simulink model "I_PD_real_ideal"  (R2018a)
settings: Solver=FixedStepAuto  StartTime=0.0  StopTime=80  RelTol=1e-3
PreLoadFcn:
  | % Parámetros de la planta
  | K0=0.82/0.017;
  | tau0=0.26;
  | N=9;
  | Kpot=1.62;
  | % Periodo de muestreo
  | Ts=0.01;
  | % Especificaciones de control deseadas
  | Sp=80; % sobreimpulso
  | Fd=0.5; % frecuencia
  | % Polos de segundo orden continuo que cumplirán las especificaciones
  | wd=2*pi*Fd ;
  | xi=sqrt((log(Sp/100))^2/(pi^2+log(Sp/100)^2))
  | wn=wd/ sqrt(1-xi^2)
  | s1=-xi*wn+j*wd
  | s2=-xi*wn-j*wd
  | % Polos de segundo orden discreto que cumpliran las especificaciones
  | p1=exp(Ts* s1 )
  | p2=exp(Ts* s2 )
  | % Insertar el tercer y cuarto polo (no dominantes)
  | p3=0.8
  | p4=0.8
  | % Función de transferencia discreta de la planta
  | Ptas=tf([K0*(1/N)*Kpot],[tau0,1,0]);
  | Ptaz=c2d(Ptas,Ts,'zoh');
  | % Coeficientes del denominador y enumerador
  | [Nz ,Dz]= tfdata(Ptaz,'v')
  | a1=Nz(2);
  | a0=Nz(3);
  | b1=Dz(2);
  | b0=Dz(3);
  | % Definiciones de las matrices A y B
  | A=[1 a1 0 0; ...
  |    b1-1 a0 a1 0;
  |    b0-b1 0 a0 a1;
  |   -b0 0 0 a0] ;
  | b=[-b1+1-p1-p2-p3-p4;
  |    -b0+b1+p1*p2-(-p1-p2)*p3-(-p1-p2-p3)*p4;
  |    b0-p1*p2*p3-(p1*p2-(-p1-p2)*p3)*p4;
  |    p1*p2*p3*p4] ;
  | % Controlador
  | x=inv(A)*b ;
  | alpha=x(1)
  | c2=x(2)
  | c1=x(3)
  | c0=x(4)
  | A2=[1 1 1; alpha-1 alpha+1 -2; -alpha alpha 1];
  | B2=[c2;c1;c0];
  | x2=inv(A2)*B2;
  | kp = x2(1)
  | ki = (2/Ts)*x2(2)
  | kd = Ts*x2(3)
undefined symbols (not defined in the file or in its folder): DiscIntNeverNeededParam
libraries: arduinolib x4, simulink x1
settings Model: SimulationMode=external  ExtModeTrigDuration=2  Creator=Eneko Lerma  LastModifiedBy=Eneko Lerma
settings SolverCC: AutoInsertRateTranBlk=on
settings OptimizationCC: EnhancedBackFolding=on  PassReuseOutputArgsAs=Individual arguments  MaxStackSize=64  OptimizeBlockOrder=speed  DifferentSizesBufferReuse=on  OptimizationCustomize=off
settings DebuggingCC: ParameterTunabilityLossMsg=error
settings HardwareCC: ProdBitPerPointer=32  ProdBitPerSizeT=32  ProdBitPerPtrDiffT=32  ProdLargestAtomicInteger=Long  ProdLargestAtomicFloat=Double  ProdWordSize=32  ProdHWDeviceType=ARM Compatible->ARM Cortex
settings SFSimCC: MATLABDynamicMemAlloc=off
settings RTWCC: SystemTargetFile=ert.tlc  HardwareBoard=Arduino Due  TLCOptions=-aInlineSetEventsForThisBaseRateFcn=TLC_FALSE -aSuppressMultiTaskScheduler=TLC_FALSE -aRateBasedStepFcn=1  TemplateMakefile=ert_default_tmf  GenerateReport=on  Toolchain=Arduino ARM  BuildConfiguration=Faster Runs  IncludeHyperlinkInReport=on  LaunchReport=on  GenerateTraceInfo=on  GenerateTraceReport=on  GenerateTraceReportSl=on  GenerateTraceReportSf=on  GenerateTraceReportEml=on
settings RTWCC: CustomTerminator=|
  | writeDigitalPin((uint8_T)3, 0);
  | writeDigitalPin((uint8_T)5, 0);
settings CodeAppCC: ForceParamTrailComments=on  IgnoreCustomStorageClasses=off  OperatorAnnotations=on  SimulinkDataObjDesc=on  SFDataObjDesc=on  InsertBlockDesc=on
settings ERTTargetCC: SupportContinuousTime=on  SupportVariableSizeSignals=on

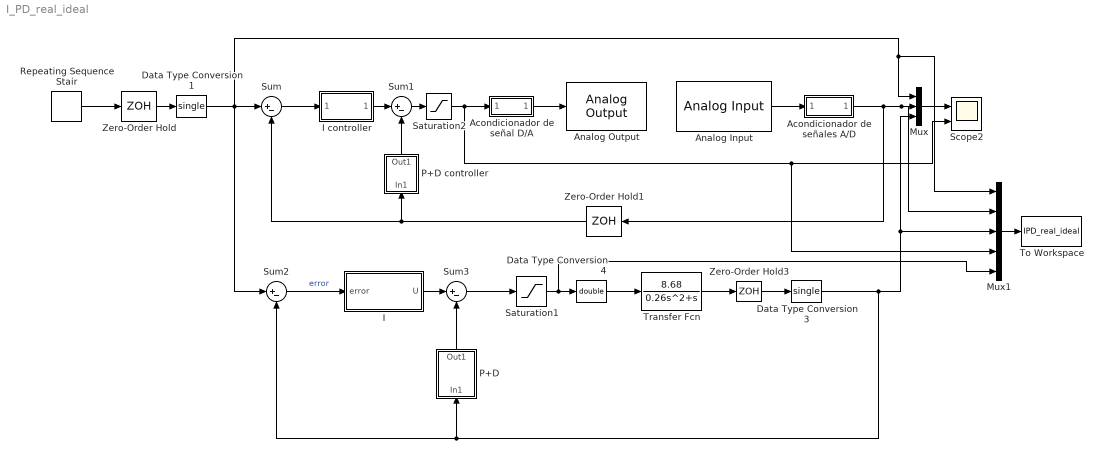
== system I_PD_real_ideal ==
  Acondicionador de señal D/A : Subsystem
  Acondicionador de señales A/D : Subsystem
  Analog Input : arduinolib/Analog Input  pinNumber=1  ReadResultsOnly=off  ConversionTriggerSource=Software  ExternalTriggerType=uint32(0)  OutputDataType=uint16  EnableConversionCompleteNotify=off  EnableOuputStatus=off  SampleTime=0.005  blockPlatform=arduino
  Analog Output : arduinolib/Analog Output  DACpin=DAC1  blockPlatform=arduino
      settings: SourceProductName=Simulink Support Package for Arduino Hardware  SourceProductBaseCode=ARDUINO
  Data Type Conversion1 : DataTypeConversion  OutDataTypeStr=single
  Data Type Conversion3 : DataTypeConversion  OutDataTypeStr=single
  Data Type Conversion4 : DataTypeConversion  OutDataTypeStr=double
  I : Subsystem
  I controller : Subsystem
  Mux : Mux  Inputs=3
  Mux1 : Mux  Inputs=5
  P+D : Subsystem
  P+D controller : Subsystem
  Repeating Sequence Stair : simulink/Sources/Repeating Sequence Stair  OutValues=[2 -2].'  tsamp=10  OutMin=[]  OutMax=[]  OutDataTypeStr=double  OutputDataTypeScalingMode=double  OutDataType=fixdt(0,8)  ConRadixGroup=Best Precision: Vector-wise  OutScaling=2^-12
  Saturation1 : Saturate  UpperLimit=5  LowerLimit=-5
  Saturation2 : Saturate  UpperLimit=5  LowerLimit=-5
  Scope2 : Scope  NumInputPorts=2
  Sum : Sum  Inputs=|+-  AccumDataTypeStr=single
  Sum1 : Sum  Inputs=|+-
  Sum2 : Sum  Inputs=|+-  AccumDataTypeStr=single
  Sum3 : Sum  Inputs=|+-  AccumDataTypeStr=single
  To Workspace : ToWorkspace  VariableName=IPD_real_ideal  SaveFormat=Structure With Time  SampleTime=-1
  Transfer Fcn : TransferFcn  Numerator=[8.68]  Denominator=[0.26 1 0]
  Zero-Order Hold : ZeroOrderHold  SampleTime=Ts
  Zero-Order Hold1 : ZeroOrderHold  SampleTime=Ts
  Zero-Order Hold3 : ZeroOrderHold  SampleTime=Ts
  wires:
  Zero-Order Hold/1 -> Data Type Conversion1/1
  I controller/1(Out1) -> Sum1/1
  Mux/1 -> Scope2/1
  P+D controller/1(Out1) -> Sum1/2
  Repeating Sequence Stair/1 -> Zero-Order Hold/1
  Acondicionador de señal D/A/1(" ") -> Analog Output/1
  Sum/1 -> I controller/1(error)
  Zero-Order Hold1/1 -> Sum/2, P+D controller/1(In1)
  Saturation2/1 -> Acondicionador de señal D/A/1("  "), Mux1/4, Scope2/2
  Analog Input/1 -> Acondicionador de señales A/D/1("  ")
  Acondicionador de señales A/D/1(" ") -> Mux1/2, Mux/2, Zero-Order Hold1/1
  Data Type Conversion4/1 -> Transfer Fcn/1
  Sum3/1 -> Saturation1/1
  Data Type Conversion3/1 -> Mux1/3, Mux/3, Sum2/2, P+D/1(In1)
  Saturation1/1 -> Mux1/5, Data Type Conversion4/1
  Zero-Order Hold3/1 -> Data Type Conversion3/1
  P+D/1(Out1) -> Sum3/2
  I/1(U) -> Sum3/1
  Transfer Fcn/1 -> Zero-Order Hold3/1
  Data Type Conversion1/1 -> Sum2/1, Mux1/1, Mux/1, Sum/1
  Sum2/1 -> I/1(error)  "error"
  Mux1/1 -> To Workspace/1
  Sum1/1 -> Saturation2/1

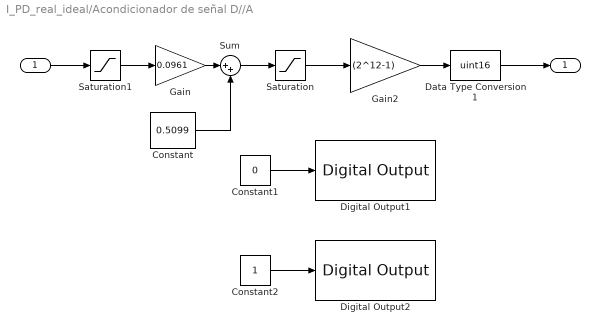
== system I_PD_real_ideal/Acondicionador de señal D//A ==
  "  " : Inport  OutDataTypeStr=single
  Constant : Constant  Value=0.5099
  Constant1 : Constant  Value=0
  Constant2 : Constant
  Data Type Conversion1 : DataTypeConversion  OutDataTypeStr=uint16
  Digital Output1 : arduinolib/Digital Output  pinNumber=5  blockPlatform=arduino
  Digital Output2 : arduinolib/Digital Output  pinNumber=3  blockPlatform=arduino
  Gain : Gain  Gain=0.0961
  Gain2 : Gain  Gain=(2^12-1)  OutDataTypeStr=single
  Saturation : Saturate  UpperLimit=1  LowerLimit=0  OutDataTypeStr=single
  Saturation1 : Saturate  UpperLimit=5  LowerLimit=-5  OutDataTypeStr=double
  Sum : Sum  Inputs=|++
  " " : Outport  OutDataTypeStr=uint16
  wires:
  Gain2/1 -> Data Type Conversion1/1
  "  "/1 -> Saturation1/1
  Sum/1 -> Saturation/1
  Data Type Conversion1/1 -> " "/1
  Saturation/1 -> Gain2/1
  Saturation1/1 -> Gain/1
  Gain/1 -> Sum/1
  Constant/1 -> Sum/2
  Constant1/1 -> Digital Output1/1
  Constant2/1 -> Digital Output2/1

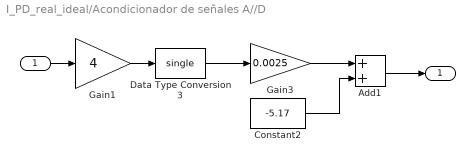
== system I_PD_real_ideal/Acondicionador de señales A//D ==
  "  " : Inport  OutDataTypeStr=uint16
  Add1 : Sum  AccumDataTypeStr=single
  Constant2 : Constant  Value=-5.17  OutDataTypeStr=single
  Data Type Conversion3 : DataTypeConversion  OutDataTypeStr=single
  Gain1 : Gain  Gain=4  OutDataTypeStr=uint16
  Gain3 : Gain  Gain=0.0025  OutDataTypeStr=single
  " " : Outport  OutDataTypeStr=single
  wires:
  Gain1/1 -> Data Type Conversion3/1
  "  "/1 -> Gain1/1
  Data Type Conversion3/1 -> Gain3/1
  Gain3/1 -> Add1/1
  Constant2/1 -> Add1/2
  Add1/1 -> " "/1

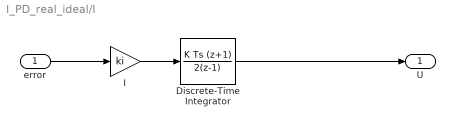
== system I_PD_real_ideal/I ==
  error : Inport
  Discrete-Time Integrator : DiscreteIntegrator  IntegratorMethod=Integration: Trapezoidal  SampleTime=Ts  ICPrevOutput=DiscIntNeverNeededParam  ICPrevScaledInput=DiscIntNeverNeededParam
  I : Gain  Gain=ki
  U : Outport  OutDataTypeStr=single
  wires:
  error/1 -> I/1
  I/1 -> Discrete-Time Integrator/1
  Discrete-Time Integrator/1 -> U/1

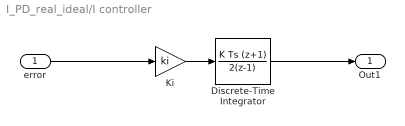
== system I_PD_real_ideal/I controller ==
  error : Inport  OutDataTypeStr=single
  Discrete-Time Integrator : DiscreteIntegrator  IntegratorMethod=Integration: Trapezoidal  SampleTime=Ts  ICPrevOutput=DiscIntNeverNeededParam  ICPrevScaledInput=DiscIntNeverNeededParam
  Ki : Gain  Gain=ki  OutDataTypeStr=single
  Out1 : Outport  OutDataTypeStr=single
  wires:
  Discrete-Time Integrator/1 -> Out1/1
  Ki/1 -> Discrete-Time Integrator/1
  error/1 -> Ki/1

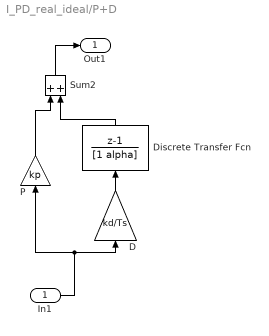
== system I_PD_real_ideal/P+D ==
  In1 : Inport
  D : Gain  Gain=kd/Ts
  Discrete Transfer Fcn : DiscreteTransferFcn  Numerator=[1 -1]  Denominator=[1 alpha]  SampleTime=Ts
  P : Gain  Gain=kp
  Sum2 : Sum
  Out1 : Outport  OutDataTypeStr=single
  wires:
  D/1 -> Discrete Transfer Fcn/1
  Discrete Transfer Fcn/1 -> Sum2/2
  P/1 -> Sum2/1
  In1/1 -> P/1, D/1
  Sum2/1 -> Out1/1

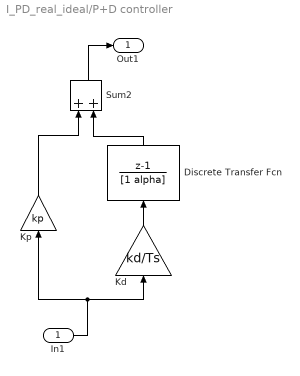
== system I_PD_real_ideal/P+D controller ==
  In1 : Inport  OutDataTypeStr=single
  Discrete Transfer Fcn : DiscreteTransferFcn  Numerator=[1 -1]  Denominator=[1 alpha]  SampleTime=Ts
  Kd : Gain  Gain=kd/Ts
  Kp : Gain  Gain=kp
  Sum2 : Sum  AccumDataTypeStr=single
  Out1 : Outport  OutDataTypeStr=single
  wires:
  Kd/1 -> Discrete Transfer Fcn/1
  In1/1 -> Kp/1, Kd/1
  Discrete Transfer Fcn/1 -> Sum2/2
  Kp/1 -> Sum2/1
  Sum2/1 -> Out1/1
